simulink model "simulinkq3"  (R2019a)
settings: Solver=VariableStepAuto  StartTime=0.0  StopTime=10.0  RelTol=1e-3
settings Model: Creator=Asus  LastModifiedBy=Asus

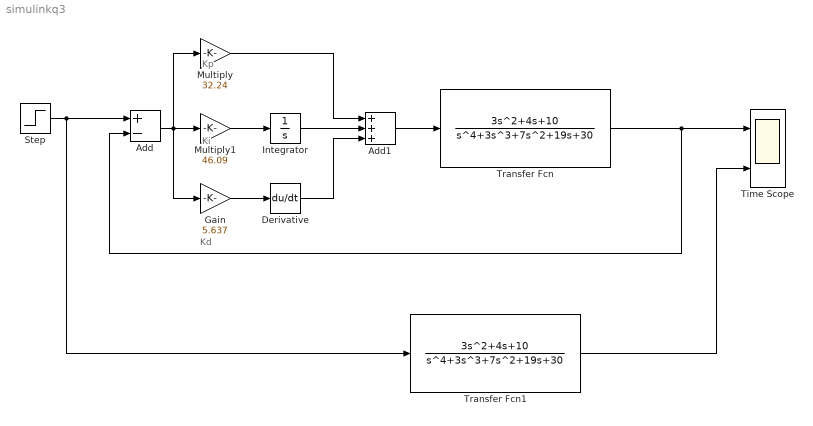
== system simulinkq3 ==
  note: Kd
  note: Ki
  note: Kp
  Add : Sum  Inputs=+-
  Add1 : Sum  Inputs=+++
  Derivative : Derivative
  Gain : Gain  Gain=5.637
  Integrator : Integrator
  Multiply : Gain  Gain=32.24
  Multiply1 : Gain  Gain=46.09
  Step : Step  SampleTime=0
  Time Scope : Scope  NumInputPorts=2
  Transfer Fcn : TransferFcn  Numerator=[3 4 10]  Denominator=[1 3 7 19 30]
  Transfer Fcn1 : TransferFcn  Numerator=[3 4 10]  Denominator=[1 3 7 19 30]
  wires:
  Transfer Fcn/1 -> Add/2, Time Scope/1
  Step/1 -> Transfer Fcn1/1, Add/1
  Add/1 -> Gain/1, Multiply/1, Multiply1/1
  Multiply1/1 -> Integrator/1
  Gain/1 -> Derivative/1
  Multiply/1 -> Add1/1
  Integrator/1 -> Add1/2
  Derivative/1 -> Add1/3
  Add1/1 -> Transfer Fcn/1
  Transfer Fcn1/1 -> Time Scope/2
